simulink model "MinJerk"  (R2025b)
settings: configuration reference "MCConfiguration" (kept outside this file)
settings Model: DataDictionary=embeddedBoard_common.sldd  Creator=rpumpo  LastModifiedBy=rpumpo
settings ConfigSetRef: SourceName=MCConfiguration

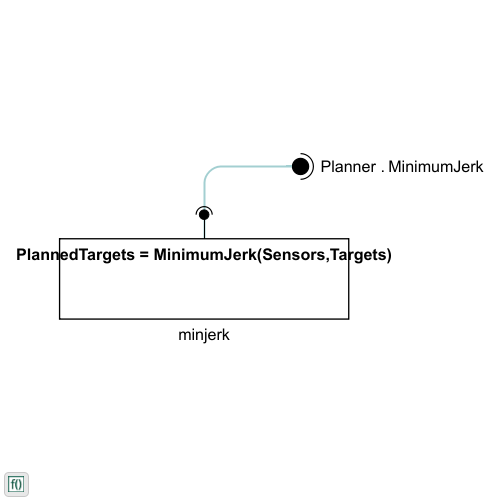
[thumbnail: Simulink's stored preview of the top-level diagram]
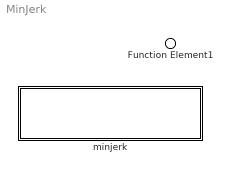
== system MinJerk ==
  minjerk : Subsystem
  Function Element1 : Outport  AllowServiceAccess=on  PortName=Planner  Element=MinimumJerk

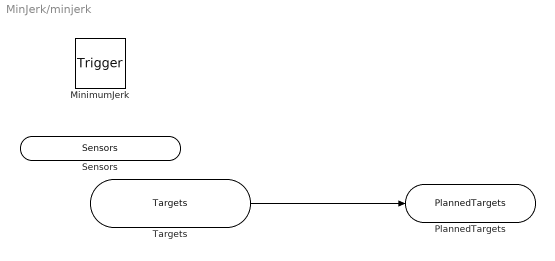
== system MinJerk/minjerk ==
  MinimumJerk : TriggerPort  TriggerType=function-call  IsSimulinkFunction=on  FunctionName=MinimumJerk  FunctionVisibility=port  ScopeName=Planner  VariantControl=(inherit)
  Sensors : ArgIn  OutDataTypeStr=single  ArgumentName=Sensors
  Targets : ArgIn  Port=2  OutDataTypeStr=Bus: Targets  ArgumentName=Targets
  PlannedTargets : ArgOut  OutDataTypeStr=Bus: Targets  ArgumentName=PlannedTargets
  wires:
  Targets/1 -> PlannedTargets/1
